simulink model "dsPIC33CK256MP508_MCLV2_SMO"  (R2021b)
settings: Solver=FixedStepDiscrete  StartTime=0.0  StopTime=10  FixedStep=.00005  RelTol=1e-3  EnableMultiTasking=on
PreLoadFcn:
  | dsPIC33CK256MP508_MCLV2_SMO_data;
InitFcn:
  | dsPIC33CK256MP508_MCLV2_SMO_data;
undefined symbols (not defined in the file): AN1, B0, B2, C9, D6, DiscIntNeverNeededParam, inverter, MaxPer, mcb_isCodeGenVar, mcb_isSimVar, P32, P57, P70, PI_params, Pin, pmsm, PU_System, PWM1max, PWM_frequency, Resol, s, Speed_openLoop, Ts, Ts_speed, us
libraries: mcbcontrolslib x13, MCHP_Blockset x13, simulink x10, mcbplantlib x1, autolibpmsmexterior x1
(part 2 of 3)

== system dsPIC33CK256MP508_MCLV2_SMO/Current Control/MOTOR Cmd ==
  PWM (abc) : Inport
  Dead time Compensation : Bias  Bias=round( (2e-6/5e-5) *PWM1max )
  Demux : Demux  Outputs=3
  PWM_HS_FEP : MCHP_Blockset/PWM IO/PWM_HS_FEP  Priority=-2000  PWMx_MODSEL=Center Aligned  PWMx_CLKSEL=no scaling  PWM_ClockResolution_DIVSEL=Dynamic Options  PWM_ClockResolution_DIVSEL_TXT=auto  PWM_ClockResolution_FSCL=Dynamic Options  PWM_ClockResolution_FSCL_TXT=auto - no jitter  PWM_ClockResolution_NoScaling=Dynamic Options  PWM_ClockResolution_NoScaling_TXT="Resol: 0.005(us)  -  MaxPer: 0.000328(s)"  MaxPeriod_s=50e-6  InitPeriode_s=50e-6  InitDutyCycleP_s=2e-6  InitDutyCycleS_s=10e-6  InitPhase_s=-1  evalin_ws=PWM1max=MCHP_Fun.Hex2num('40B3880000000000');PWM2max=MCHP_Fun.Hex2num('40B3880000000000');PWM3max=MCHP_Fun.Hex2num('40B3880000000000');  SampleTime=-1  S_INPUT=[-1]  S_INPUT_Size=[3]  S_OUTPUT=[]  S_OUTPUT_Size=[]  S_ListCustomDatatype=S.S_ListCustomDatatype={};  MCHP_USER_INTERRUPTS=0  MCHP_PORT={PWMH1 }{PWMH1}32:4:B14;{PWMH2 }{PWMH2}32:4:B12;{PWMH3 }{PWMH3}32:4:B10;{PWML1}{PWML1}32:4:B15;{PWML2}{PWML2}32:4:B13;{PWML3}{PWML3}32:4:B11;  MCHP_MASTERLINK=dsPIC33CK256MP508_MCLV2_SMO1/Hardware Init/Microchip Master  MCHP_CRC=4827838  PWMx_PMOD=Complementary  PWM1_HL=PWMxH & PWMxL output enabled  PWM1_swap=off  PWM1H_pol=off  PWM1L_pol=off  PWM2_HL=PWMxH & PWMxL output enabled  PWM2_swap=off  PWM2H_pol=off  PWM2L_pol=off  PWM3_HL=PWMxH & PWMxL output enabled  PWM3_swap=off  PWM3H_pol=off  PWM3L_pol=off  PWM4_HL=not used  PWM4_swap=off  PWM4H_pol=off  PWM4L_pol=off  PWM5_HL=not used  PWM5_swap=off  PWM5H_pol=off  PWM5L_pol=off  PWM6_HL=not used  PWM6_swap=off  PWM6H_pol=off  PWM6L_pol=off  PWM7_HL=not used  PWM7_swap=off  PWM7H_pol=off  PWM7L_pol=off  PWM8_HL=not used  PWM8_swap=off  PWM8H_pol=off  PWM8L_pol=off  PWM9_HL=not used  PWM9_swap=off  PWM9H_pol=off  PWM9L_pol=off  PWM10_HL=not used  PWM10_swap=off  PWM10H_pol=off  PWM10L_pol=off  PWM11_HL=not used  PWM11_swap=off  PWM11H_pol=off  PWM11L_pol=off  PWM12_HL=not used  PWM12_swap=off  PWM12H_pol=off  PWM12L_pol=off  PWM1_ShowTrig=on  PWM1_Init_PGxTRIGABC_s=[0 -1 -1 ]  PWM1_ADTRxEN1=ADC Trigger 1  PWM1_ADTRxEN2=none  PWM1_ADTRxEN3=none  PWM2_ShowTrig=off  PWM2_Init_PGxTRIGABC_s=[-1 -1 -1]  PWM2_ADTRxEN1=none  PWM2_ADTRxEN2=none  PWM2_ADTRxEN3=none  PWM3_ShowTrig=off  PWM3_Init_PGxTRIGABC_s=[-1 -1 -1]  PWM3_ADTRxEN1=none  PWM3_ADTRxEN2=none  PWM3_ADTRxEN3=none  PWM4_ShowTrig=off  PWM4_Init_PGxTRIGABC_s=[-1 -1 -1]  PWM4_ADTRxEN1=none  PWM4_ADTRxEN2=none  PWM4_ADTRxEN3=none  PWM5_ShowTrig=off  PWM5_Init_PGxTRIGABC_s=[-1 -1 -1]  PWM5_ADTRxEN1=none  PWM5_ADTRxEN2=none  PWM5_ADTRxEN3=none  PWM6_ShowTrig=off  PWM6_Init_PGxTRIGABC_s=[-1 -1 -1]  PWM6_ADTRxEN1=none  PWM6_ADTRxEN2=none  PWM6_ADTRxEN3=none  PWM7_ShowTrig=off  PWM7_Init_PGxTRIGABC_s=[-1 -1 -1]  PWM7_ADTRxEN1=none  PWM7_ADTRxEN2=none  PWM7_ADTRxEN3=none  PWM8_ShowTrig=off  PWM8_Init_PGxTRIGABC_s=[-1 -1 -1]  PWM8_ADTRxEN1=none  PWM8_ADTRxEN2=none  PWM8_ADTRxEN3=none  BlockInput_VectorScalar=Independant Scalar  BlockInput_Period=Not a block input  BlockInput_DutyCycle=a Uint raw input (PWMxmax variable represent max period)  BlockInput_PhaseShift=Not a block input  BlockInput_SEVTCMP=Not a block input  BlockInput_TRIGx=Not a block input  BlockInput_DeadTime=Not a block input  BlockOutput_FaultDisabled=off  BlockOutput_Fault=on  DTC=Positive dead time (ensure period of time with PWM_H and PWM_L disasserted)  FLTSRC1_DTCMP=Dynamic Options  FLTSRC1_DTCMP_TXT=<empty>  FLTSRC2_DTCMP=Dynamic Options  FLTSRC2_DTCMP_TXT=<empty>  FLTSRC3_DTCMP=Dynamic Options  FLTSRC3_DTCMP_TXT=<empty>  FLTSRC4_DTCMP=Dynamic Options  FLTSRC4_DTCMP_TXT=<empty>  FLTSRC5_DTCMP=Dynamic Options  FLTSRC5_DTCMP_TXT=<empty>  FLTSRC6_DTCMP=Dynamic Options  FLTSRC6_DTCMP_TXT=<empty>  FLTSRC7_DTCMP=Dynamic Options  FLTSRC7_DTCMP_TXT=<empty>  FLTSRC8_DTCMP=Dynamic Options  FLTSRC8_DTCMP_TXT=<empty>  FLTSRC9_DTCMP=Dynamic Options  FLTSRC9_DTCMP_TXT=<empty>  FLTSRC10_DTCMP=Dynamic Options  FLTSRC10_DTCMP_TXT=<empty>  FLTSRC11_DTCMP=Dynamic Options  FLTSRC11_DTCMP_TXT=<empty>  FLTSRC12_DTCMP=Dynamic Options  FLTSRC12_DTCMP_TXT=<empty>  DeadTime_s=1e-6  DeadTimeAlt_s=1e-6  DeadTimeComp_s=0  FLTMODx=Disabled  FLTSRCx=Dynamic Options  FLTSRCx_TXT=<empty>  FLTDATx=PWM H/L -> 11  CLMODx=Disabled  CLSRCx=Dynamic Options  CLSRCx_TXT=<empty>  CLDATx=PWM H/L -> 00  FLTLEBENx=off  CLLEBENx=off  LeadEdgeBlkPer_s=5e-7  PHRx=off  PHFx=off  PLRx=off  PLFx=off
      settings: SourceProductName=MPLAB Device Blocks for Simulink
  "Saturation " : Saturate  UpperLimit=PWM1max  LowerLimit=round( (2e-6/5e-5) *PWM1max )* 2
  int to uint : DataTypeConversion  OutDataTypeStr=uint16  ConvertRealWorld=Stored Integer (SI)
  tag scope: Duty1=global
  wires:
  int to uint/1 -> "Saturation "/1
  Dead time Compensation/1 -> [Duty1], int to uint/1
  PWM (abc)/1 -> Dead time Compensation/1
  "Saturation "/1 -> Demux/1
  Demux/2 -> PWM_HS_FEP/2
  Demux/3 -> PWM_HS_FEP/3
  Demux/1 -> PWM_HS_FEP/1

== system dsPIC33CK256MP508_MCLV2_SMO/Current Control/MOTOR - Board Sensor ==
  ADC dsPIC High Speed SAR : MCHP_Blockset/Analog IO/ADC dsPIC High Speed SAR  ACLKCON=Not used  ADC_FRACT=Fractional (left aligned)  ADC_NRE=off  DMA_Size=Single trigger - (default)  ADC_Synchronisation=Triggered by custom source  ADC_Trig=Dynamic Options  ADC_Trig_TXT=PWM1 Trigger 1  ADC_TrigTimeStep=Trig model step after all sample from this block are converted  ADC_TrigInfo=0  SampleTime=Ts  S_INPUT=[]  S_INPUT_Size=[]  S_OUTPUT="[5  5]"  S_OUTPUT_Size="[1  1]"  S_ListCustomDatatype=S.S_ListCustomDatatype={};  MCHP_USER_INTERRUPTS={ADCAN1}{ADCBUF1}{ADC Data 1 Ready}{VectorName(ADCAN1Interrupt) Priority(-1) RegisterReadClear(ADCBUF1)Config_BitSet(ADIELbits.IE1) };{ADCAN3}{ADCBUF3}{ADC Data 3 Ready}{VectorName(ADCAN3Interrupt) Priority(-1) RegisterReadClear(ADCBUF3)Config_BitSet(ADIELbits.IE3) };{ADCAN18}{ADCBUF18}{ADC Data 18 Ready}{VectorName(ADCAN18Interrupt) Priority(-1) RegisterReadClear(ADCBUF18)Config_BitSet(ADIEHbits.IE18) };  MCHP_PORT={Analog Input 1}{AN1}15:2:B2;{Analog Input 4}{AN4}15:2:A4;{Analog Input 19}{AN19}15:2:D11;  MCHP_MASTERLINK=dsPIC33CK256MP508_MCLV2_SMO1/Hardware Init/Microchip Master  MCHP_CRC=4003151  ADC_Info=Total Time = 4.92(us)  ADC0_pin=Dynamic Options  ADC0_pin_TXT=Not used  ADC0_R="< 50   kOhm"  ADC0_res=12 bits  ADC0_signed=signed 16 bits  ADC0_FILTER=No Oversampling  ADC0_FILTER_nSamples=256 samples  ADC0_STRGEN=Start sampling followed by conversion  ADC0_STRGEN_on=Start sampling followed by conversion  ADC0_SSAMPEN=off  ADC0_Info=tSmp_min=20(ns) x 0 = 0(s) ; tConv=210(ns) x 0 = 0(s) ; TOTAL=0(s)  ADC1_pin=Dynamic Options  ADC1_pin_TXT=AN1 / B2 / Pin[41]  ADC1_R="< 50   kOhm"  ADC1_res=12 bits  ADC1_signed=signed 16 bits  ADC1_FILTER=No Oversampling  ADC1_FILTER_nSamples=128 samples  ADC1_STRGEN=Start sampling followed by conversion  ADC1_STRGEN_on=Start sampling followed by conversion  ADC1_SSAMPEN=off  ADC1_Info=tSmp_min=2.06(us) x 1 = 2.06(us) ; tConv=370(ns) x 1 = 370(ns) ; TOTAL=2.44(us)  ADC2_pin=Dynamic Options  ADC2_pin_TXT=Not used  ADC2_R="< 5    kOhm"  ADC2_res=12 bits  ADC2_signed=signed 16 bits  ADC2_FILTER=No Oversampling  ADC2_FILTER_nSamples=256 samples  ADC2_STRGEN=End sampling and start conversion  ADC2_STRGEN_on=Start sampling followed by conversion  ADC2_SSAMPEN=on  ADC2_Info=tSmp_min=14.706(ns) x 0 = 0(s) ; tConv=154.41(ns) x 0 = 0(s) ; TOTAL=0(s)  ADC3_pin=Dynamic Options  ADC3_pin_TXT=Not used  ADC3_R="< 10   kOhm"  ADC3_res=12 bits  ADC3_signed=signed 16 bits  ADC3_FILTER=Burst convert of n samples are Summed  ADC3_FILTER_nSamples=64 samples  ADC3_STRGEN=End sampling and start conversion  ADC3_STRGEN_on=Start sampling followed by conversion  ADC3_SSAMPEN=on  ADC3_Info=tSmp_min=14.706(ns) x 0 = 0(s) ; tConv=154.41(ns) x 0 = 0(s) ; TOTAL=0(s)  ADC4_pin=Dynamic Options  ADC4_pin_TXT=Not used  ADC4_R=< 200 Ohm  ADC4_res=12 bits  ADC4_signed=unsigned 16 bits  ADC4_FILTER=No Oversampling  ADC4_FILTER_nSamples=256 samples  ADC4_STRGEN=End sampling and start conversion  ADC4_STRGEN_on=Start sampling followed by conversion  ADC4_SSAMPEN=off  ADC4_Info=tSmp_min=14.706(ns) x 0 = 0(s) ; tConv=154.41(ns) x 0 = 0(s) ; TOTAL=0(s)  ADC5_pin=Dynamic Options  ADC5_pin_TXT=Not used  ADC5_R=< 200 Ohm  ADC5_res=12 bits  ADC5_signed=unsigned 16 bits  ADC5_FILTER=Burst convert of n samples are Summed  ADC5_FILTER_nSamples=256 samples  ADC5_STRGEN=End sampling and start conversion  ADC5_STRGEN_on=Start sampling followed by conversion  ADC5_SSAMPEN=on  ADC5_Info=tSmp_min=14.706(ns) x 0 = 0(s) ; tConv=154.41(ns) x 0 = 0(s) ; TOTAL=0(s)  ADC6_pin=Dynamic Options  ADC6_pin_TXT=Not used  ADC6_R=< 200 Ohm  ADC6_res=12 bits  ADC6_signed=unsigned 16 bits  ADC6_FILTER=Burst convert of n samples are Summed  ADC6_FILTER_nSamples=256 samples  ADC6_STRGEN=End sampling and start conversion  ADC6_STRGEN_on=Start sampling followed by conversion  ADC6_SSAMPEN=on  ADC6_Info=tSmp_min=14.706(ns) x 0 = 0(s) ; tConv=154.41(ns) x 0 = 0(s) ; TOTAL=0(s)  ADC7_R="< 50   kOhm"  ADC7_res=12 bits  ADC7_AN0=Not used  ADC7_AN1=Not used  ADC7_AN2=Not used  ADC7_AN3=Not used  ADC7_AN4=signed int16  ADC7_AN5=Not used  ADC7_AN6=Not used  ADC7_AN7=Not used  ADC7_AN8=Not used  ADC7_AN9=Not used  ADC7_AN10=Not used  ADC7_AN11=Not used  ADC7_AN12=Not used  ADC7_AN13=Not used  ADC7_AN14=Not used  ADC7_AN15=Not used  ADC7_AN16=Not used  ADC7_AN17=Not used  ADC7_AN18=Not used  ADC7_AN19=unsigned int16  ADC7_AN20=Not used  ADC7_AN21=Not used  ADC7_AN22=Not used  ADC7_AN23=Not used  ADC7_AN24=Not used  ADC7_AN25=Not used  ADC7_AN26=Not used  ADC7_AN27=Not used  ADC7_AN28=Not used  ADC7_AN29=Not used  ADC7_AN30=Not used  ADC7_AN31=Not used  IVref=Not used  IVTemp=Not used  ADC7_Info=tSmp_min=2.08(us) x 2 = 4.16(us) ; tConv=370(ns) x 2 = 740(ns) ; TOTAL=4.92(us)
      settings: SourceProductName=MPLAB Device Blocks for Simulink
  Add2 : Sum  Inputs=+-  OutDataTypeStr=int16  RndMeth=Simplest
  Data Store Read : DataStoreRead  DataStoreName=EnCurOffset  IndexOptions=Index vector (dialog)  Indices=1  OutputSizes=1
  Data Type Conversion : DataTypeConversion  OutDataTypeStr=dataType  RndMeth=Simplest
  Gain Correction : Subsystem
  Mux2 : Mux  Inputs=2
  Offset1 : Subsystem
  Q1.15 : DataTypeConversion  OutDataTypeStr=fixdt(0,16,16)  ConvertRealWorld=Stored Integer (SI)
  Scale Ia Ib to (A) : DataTypeConversion  OutDataTypeStr=fixdt(1,16, 1.65/32768 / (.005 * 75),0)  ConvertRealWorld=Stored Integer (SI)
  Pot : Outport  VectorParamsAs1DForOutWhenUnconnected=off
  Iab (A) : Outport  Port=2  VectorParamsAs1DForOutWhenUnconnected=off
  tag scope: Iab=global, Pot=global
  wires:
  Mux2/1 -> Add2/1, Offset1/1(Iab)
  ADC dsPIC High Speed SAR/3 -> Q1.15/1  "U2 CH2"
  Q1.15/1 -> Data Type Conversion/1
  Scale Ia Ib to (A)/1 -> Gain Correction/1(In1)  "Ia Ib"
  Offset1/1(Offset) -> Add2/2
  Add2/1 -> Scale Ia Ib to (A)/1
  Data Store Read/1 -> Offset1/Enable
  Data Type Conversion/1 -> Pot/1, [Pot]
  Gain Correction/1(Out1) -> Iab (A)/1, [Iab]
  ADC dsPIC High Speed SAR/1 -> Mux2/1
  ADC dsPIC High Speed SAR/2 -> Mux2/2

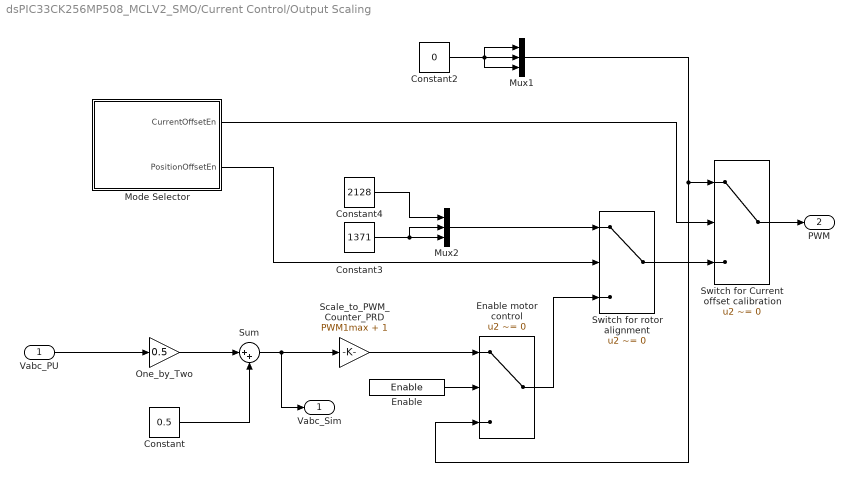
== system dsPIC33CK256MP508_MCLV2_SMO/Current Control/Output Scaling ==
  Vabc_PU : Inport
  Constant : Constant  Value=0.5  OutDataTypeStr=dataType  SampleTime=-1
  Constant2 : Constant  Value=0  OutDataTypeStr=Inherit: Inherit via back propagation
  Constant3 : Constant  Value=1371  OutDataTypeStr=Inherit: Inherit via back propagation
  Constant4 : Constant  Value=2128  OutDataTypeStr=Inherit: Inherit via back propagation
  Enable : DataStoreRead  DataStoreName=Enable  IndexOptions=Index vector (dialog)  Indices=1  OutputSizes=1
  Enable motor control : Switch  Criteria=u2 ~= 0  Threshold=250
  Mode Selector : Subsystem
  Mux1 : Mux  Inputs=3
  Mux2 : Mux  Inputs=3
  One_by_Two : Gain  Gain=0.5  RndMeth=Simplest  OutDataTypeStr=Inherit: Same as input
  Scale_to_PWM_Counter_PRD : Gain  Gain=PWM1max + 1  OutDataTypeStr=uint16  RndMeth=Simplest
  Sum : Sum  Inputs=|++
  Switch for Current offset calibration : Switch  Criteria=u2 ~= 0  Threshold=250
  Switch for rotor alignment : Switch  Criteria=u2 ~= 0  Threshold=250
  Vabc_Sim : Outport
  PWM : Outport  Port=2
  wires:
  Sum/1 -> Scale_to_PWM_Counter_PRD/1, Vabc_Sim/1
  Constant/1 -> Sum/2
  Switch for Current offset calibration/1 -> PWM/1
  One_by_Two/1 -> Sum/1
  Switch for rotor alignment/1 -> Switch for Current offset calibration/3
  Scale_to_PWM_Counter_PRD/1 -> Enable motor control/1
  Vabc_PU/1 -> One_by_Two/1
  Mode Selector/2(PositionOffsetEn) -> Switch for rotor alignment/2
  Mux2/1 -> Switch for rotor alignment/1
  Mux1/1 -> Enable motor control/3, Switch for Current offset calibration/1
  Constant2/1 -> Mux1/1, Mux1/3, Mux1/2
  Constant3/1 -> Mux2/3, Mux2/2
  Constant4/1 -> Mux2/1
  Mode Selector/1(CurrentOffsetEn) -> Switch for Current offset calibration/2
  Enable/1 -> Enable motor control/2
  Enable motor control/1 -> Switch for rotor alignment/3

== system dsPIC33CK256MP508_MCLV2_SMO/Current Control/Serial Tx ==
  Data : Inport
  Counter Limited : simulink/Sources/Counter Limited  uplimit=3  tsamp=-1
  Data Type Conversion : DataTypeConversion  OutDataTypeStr=uint8  RndMeth=Simplest
  Demux : Demux
  Index Vector : MultiPortSwitch  DataPortOrder=Zero-based contiguous  Inputs=4  zeroidx=on  OutDataTypeStr=Inherit: Same as first data input  RndMeth=Simplest
  UART_TX : Subsystem
  wires:
  Data Type Conversion/1 -> UART_TX/1(Count), Index Vector/1
  Index Vector/1 -> UART_TX/2(Data)
  Demux/4 -> Index Vector/5
  Demux/3 -> Index Vector/4
  Demux/1 -> Index Vector/2
  Demux/2 -> Index Vector/3
  Data/1 -> Demux/1
  Counter Limited/1 -> Data Type Conversion/1

== system dsPIC33CK256MP508_MCLV2_SMO/Hardware Init/Open Board and Motor pages ==

== system dsPIC33CK256MP508_MCLV2_SMO/Inverter and Motor/Codegeneration ==
  Duty_Cycles : Inport
  Ground : Ground
  Terminator : Terminator
  Feedbacks_Iab : Outport  VectorParamsAs1DForOutWhenUnconnected=off
  wires:
  Ground/1 -> Feedbacks_Iab/1
  Duty_Cycles/1 -> Terminator/1

== system dsPIC33CK256MP508_MCLV2_SMO/Inverter and Motor/Simulation ==
  Duty_Cycles : Inport
  Gain9 : Gain  Gain=(60/(2*pi))/PU_System.N_base
  Inverter : Subsystem
  Load_Profile (Torque) : Subsystem
  Scope : Scope
  Scope1 : Scope
  Scope2 : Scope
  Sensor_Measurements : Subsystem
  Surface Mount PMSM : autolibpmsmexterior/Surface Mount PMSM  port_config=Torque  sim_type=Discrete  Ts=Ts  P=pmsm.p  Rs=pmsm.Rs + inverter.R_board  Ldq_=pmsm.Ld  KConstText=Permanent flux linkage constant (lambda_pm):  lambda_pm=pmsm.FluxPM  Ke=159.9771  Kt=1.323  mechanical=[pmsm.J, pmsm.B, 0]  idq0=[0 0]  theta_init=0  omega_init=0  KConst=pmsm.FluxPM  lambda_pm_calc=pmsm.FluxPM  RefBlkName='autolibpmsmexterior/Surface Mount PMSM'  aMode=5  Ldq="[0.0002      0.0002]"
      settings: SourceProductBaseCode=PW,DR,MT,UV,VE
  Terminator : Terminator
  Terminator1 : Terminator
  Feedbacs_Iab : Outport  VectorParamsAs1DForOutWhenUnconnected=off
  wires:
  Surface Mount PMSM/1 -> Sensor_Measurements/1(Info)
  Duty_Cycles/1 -> Scope2/1, Inverter/1(Duty_abc)
  Surface Mount PMSM/2 -> Sensor_Measurements/2(PhaseCurr)  "Iabc"
  Sensor_Measurements/1(Iab_fb) -> Scope/1, Feedbacs_Iab/1
  Load_Profile (Torque)/1(Load_Trq) -> Surface Mount PMSM/1
  Inverter/1(Vabc) -> Scope1/1, Surface Mount PMSM/2
  Sensor_Measurements/2(Pos_fb) -> Terminator1/1
  Gain9/1 -> Terminator/1
  Surface Mount PMSM/3 -> Gain9/1

== system dsPIC33CK256MP508_MCLV2_SMO/Speed Control/Enable Switch ==
  Codegen : Subsystem  VariantControl=mcb_isCodeGenVar()
  Sim : Subsystem  VariantControl=mcb_isSimVar()

== system dsPIC33CK256MP508_MCLV2_SMO/Speed Control/PI_Controller_Speed ==
  N_ref : Inport
  N_fb : Inport  Port=2
  Data Store Read1 : DataStoreRead  DataStoreName=EnSpeedCtrl  IndexOptions=Index vector (dialog)  Indices=1  OutputSizes=1
  Discrete PI Controller with anti-windup & reset : mcbcontrolslib/Discrete PI Controller  with anti-windup & reset  UpperSaturationLimit=1  LowerSaturationLimit=-1
      settings: SourceProductBaseCode=MT
  Ki1 : Constant  Value=PI_params.Ki_speed*Ts_speed  OutDataTypeStr=dataType  SampleTime=-1
  Ki2 : Constant  Value=0  OutDataTypeStr=dataType  SampleTime=-1
  Kp1 : Constant  Value=PI_params.Kp_speed  OutDataTypeStr=dataType  SampleTime=-1
  Logical Operator : Logic  Operator=NOT  IconShape=distinctive  AllPortsSameDT=off  OutDataTypeStr=boolean
  Scope : Scope
  Sum : Sum  Inputs=|+-  OutDataTypeStr=Inherit: Same as first input
  Zero_Cancellation : mcbcontrolslib/IIR Filter  VariantControl=Low Pass Filter  VariantSelect=Low-pass  Filter_constant=0.001*(Ts_speed/Ts)  advancedSettings=off  Ts=50e-6  cutOff_freq=98.4464
      settings: SourceProductBaseCode=MT
  Iq_ref : Outport  VectorParamsAs1DForOutWhenUnconnected=off
  wires:
  Discrete PI Controller with anti-windup & reset/1 -> Iq_ref/1
  Ki1/1 -> Discrete PI Controller with anti-windup & reset/3
  Kp1/1 -> Discrete PI Controller with anti-windup & reset/2
  N_fb/1 -> Sum/2
  N_ref/1 -> Zero_Cancellation/1
  Sum/1 -> Discrete PI Controller with anti-windup & reset/1
  Logical Operator/1 -> Scope/1, Discrete PI Controller with anti-windup & reset/4
  Ki2/1 -> Discrete PI Controller with anti-windup & reset/5
  Data Store Read1/1 -> Logical Operator/1
  Zero_Cancellation/1 -> Sum/1

== system dsPIC33CK256MP508_MCLV2_SMO/Speed Control/Speed_Ref_Selector ==
  Speed_Ref_In : Inport
  Constant : Constant  Value=0  OutDataTypeStr=dataType
  Data Store Read1 : DataStoreRead  DataStoreName=EnableFOC  IndexOptions=Index vector (dialog)  Indices=1  OutputSizes=1
  Switch : Switch  Criteria=u2 > Threshold  Threshold=0.5
  Speed_Ref_PU : Outport
  wires:
  Switch/1 -> Speed_Ref_PU/1
  Constant/1 -> Switch/3
  Speed_Ref_In/1 -> Switch/1
  Data Store Read1/1 -> Switch/2

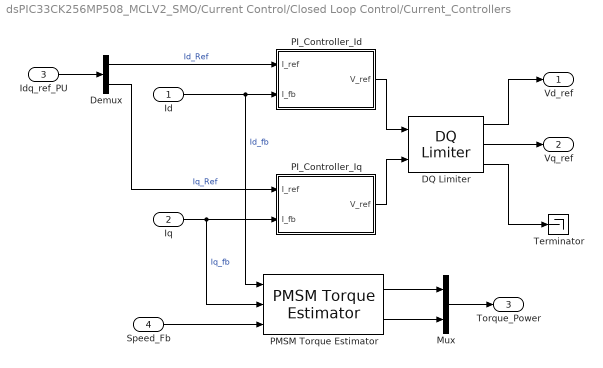
== system dsPIC33CK256MP508_MCLV2_SMO/Current Control/Closed Loop Control/Current_Controllers ==
  Id : Inport
  Iq : Inport  Port=2
  Idq_ref_PU : Inport  Port=3
  Speed_Fb : Inport  Port=4
  DQ Limiter : mcbcontrolslib/DQ Limiter  Vmax=0.95
      settings: SourceProductBaseCode=MT
  Demux : Demux  Outputs=2
  Mux : Mux  Inputs=2
  PI_Controller_Id : Subsystem
  PI_Controller_Iq : Subsystem
  PMSM Torque Estimator : mcbcontrolslib/PMSM Torque Estimator  polePairs=pmsm.p  Ld=pmsm.Ld  Lq=pmsm.Lq  FluxPM=pmsm.FluxPM  Units=Per-Unit (PU)  V_base=PU_System.V_base  I_base=PU_System.I_base  N_base=PU_System.N_base  T_base=0.26718  P_base=91.4523
      settings: SourceProductBaseCode=MT
  Terminator : Terminator
  Vd_ref : Outport  VectorParamsAs1DForOutWhenUnconnected=off
  Vq_ref : Outport  Port=2  VectorParamsAs1DForOutWhenUnconnected=off
  Torque_Power : Outport  Port=3
  wires:
  Iq/1 -> PMSM Torque Estimator/2, PI_Controller_Iq/2(I_fb)  "Iq_fb"
  Id/1 -> PMSM Torque Estimator/1, PI_Controller_Id/2(I_fb)  "Id_fb"
  Demux/1 -> PI_Controller_Id/1(I_ref)  "Id_Ref"
  Demux/2 -> PI_Controller_Iq/1(I_ref)  "Iq_Ref"
  Idq_ref_PU/1 -> Demux/1
  PI_Controller_Id/1(V_ref) -> DQ Limiter/1
  PI_Controller_Iq/1(V_ref) -> DQ Limiter/2
  DQ Limiter/1 -> Vd_ref/1
  DQ Limiter/2 -> Vq_ref/1
  DQ Limiter/3 -> Terminator/1
  PMSM Torque Estimator/1 -> Mux/1
  PMSM Torque Estimator/2 -> Mux/2
  Mux/1 -> Torque_Power/1
  Speed_Fb/1 -> PMSM Torque Estimator/3

== system dsPIC33CK256MP508_MCLV2_SMO/Current Control/Input Scaling/OpenLoopTheta ==
  Enable : EnablePort
  Constant : Constant  Value=500/PU_System.N_base  OutDataTypeStr=dataType
  Data Type Conversion : DataTypeConversion  OutDataTypeStr=fixdt(1,32,20)  ConvertRealWorld=Stored Integer (SI)
  Discrete-Time Integrator : DiscreteIntegrator  IntegratorMethod=Accumulation: Forward Euler  gainval=0.002  SampleTime=Ts  OutDataTypeStr=fixdt(1,32,20)  LimitOutput=on  UpperSaturationLimit=500/PU_System.N_base  LowerSaturationLimit=0  ICPrevOutput=DiscIntNeverNeededParam  ICPrevScaledInput=DiscIntNeverNeededParam
  Gain : Gain  Gain=Ts*PU_System.N_base*pmsm.p/60  OutDataTypeStr=dataType  ParamDataTypeStr=Inherit: Same as input
  Position Generator : mcbcontrolslib/Position Generator  AngleOutput=Per-unit  ThetaSource=External  ThetaInput=5e-4  DataType=double  ExternalReset=none  Offset=0
      settings: SourceProductBaseCode=MT
  Scope : Scope
  eps : Outport
  wires:
  Gain/1 -> Position Generator/1
  Constant/1 -> Data Type Conversion/1
  Data Type Conversion/1 -> Discrete-Time Integrator/1
  Position Generator/1 -> Scope/1, eps/1
  Discrete-Time Integrator/1 -> Gain/1

== system dsPIC33CK256MP508_MCLV2_SMO/Current Control/Input Scaling/OpentoClosed ==
  Speed_fb : Inport
  Chart : Stateflow chart  TreatAsAtomicUnit=on
  Data Store Read5 : DataStoreRead  DataStoreName=Enable  IndexOptions=Index vector (dialog)  Indices=1  OutputSizes=1
  Data Store Write1 : DataStoreWrite  DataStoreName=EnSpeedCtrl  IndexOptions=Index vector (dialog)  Indices=1  OutputSizes=1
  Data Store Write2 : DataStoreWrite  DataStoreName=EnableClosedLoop  IndexOptions=Index vector (dialog)  Indices=1  OutputSizes=1
  Data Type Conversion : DataTypeConversion  OutDataTypeStr=boolean  RndMeth=Simplest
  Data Type Conversion1 : DataTypeConversion  OutDataTypeStr=boolean
  Enable Closed Loop : Constant  OutDataTypeStr=uint16
  Enable Closed Loop1 : Constant  Value=Speed_openLoop/PU_System.N_base  OutDataTypeStr=dataType
  Open Loop Start-up : Constant  Value=0  OutDataTypeStr=uint16
  Switch2 : Switch  Criteria=u2 > Threshold  Threshold=1
  EnClosedLoop : Outport
  wires:
  Open Loop Start-up/1 -> Switch2/3
  Data Store Read5/1 -> Chart/3(En)
  Chart/1(Mode) -> Switch2/2
  Switch2/1 -> Data Type Conversion/1
  Speed_fb/1 -> Chart/2(SpeedFb)
  Enable Closed Loop/1 -> Switch2/1
  Enable Closed Loop1/1 -> Chart/1(Limit)
  Data Type Conversion/1 -> EnClosedLoop/1, Data Store Write2/1
  Chart/2(SpeedCtrl) -> Data Type Conversion1/1
  Data Type Conversion1/1 -> Data Store Write1/1

== system dsPIC33CK256MP508_MCLV2_SMO/Current Control/Input Scaling/Sliding Mode Observer ==
  Ialpha_PU : Inport
  Ibeta_PU : Inport  Port=2
  Valpha_PU : Inport  Port=3
  Vbeta_PU : Inport  Port=4
  SpeedRef_PU : Inport  Port=5
  Scaling : Subsystem
  smo : Subsystem
  theta : Outport
  west : Outport  Port=2
  wires:
  Scaling/1(Ialpha) -> smo/1(ialfa)
  Scaling/5(SpeedRef) -> smo/5(wref)
  Valpha_PU/1 -> Scaling/3(Valpha_PU)
  Scaling/4(Vbeta) -> smo/4(vbeta)
  Scaling/2(Ibeta) -> smo/2(ibeta)
  Scaling/3(Valpha) -> smo/3(valfa)
  smo/2(west) -> west/1
  SpeedRef_PU/1 -> Scaling/5(SpeedRef_PU)
  smo/1(theta) -> theta/1
  Vbeta_PU/1 -> Scaling/4(Vbeta_PU)
  Ibeta_PU/1 -> Scaling/2(Ibeta_PU)
  Ialpha_PU/1 -> Scaling/1(Ialpha_PU)

== system dsPIC33CK256MP508_MCLV2_SMO/Current Control/MOTOR - Board Sensor/Gain Correction ==
  In1 : Inport
  Demux : Demux  Outputs=2
  Gain : Gain  Gain=0.865  RndMeth=Zero  OutDataTypeStr=Inherit: Same as input
  Gain1 : Gain  Gain=0.961  RndMeth=Zero  OutDataTypeStr=Inherit: Same as input
  Mux : Mux  Inputs=2
  To Per-Unit : Gain  Gain=inverter.invertingAmp/PU_System.I_base  OutMin=-1  OutMax=1  OutDataTypeStr=fixdt(1,16)  RndMeth=Zero
  Out1 : Outport
  wires:
  Demux/1 -> Gain/1
  To Per-Unit/1 -> Demux/1
  Gain/1 -> Mux/1
  Mux/1 -> Out1/1
  In1/1 -> To Per-Unit/1
  Demux/2 -> Gain1/1
  Gain1/1 -> Mux/2

== system dsPIC33CK256MP508_MCLV2_SMO/Current Control/MOTOR - Board Sensor/Offset1 ==
  Iab : Inport
  Enable : EnablePort
  Offset : Outport
  wires:
  Iab/1 -> Offset/1

== system dsPIC33CK256MP508_MCLV2_SMO/Current Control/Output Scaling/Mode Selector ==
  Delay : Delay  DelayLength=1
  NOT : Logic  Operator=NOT  IconShape=distinctive  AllPortsSameDT=off  OutDataTypeStr=boolean
  Subsystem1 : Subsystem
  Up Counter : Subsystem
  CurrentOffsetEn : Outport
  PositionOffsetEn : Outport  Port=2
  wires:
  Up Counter/1(Count) -> Subsystem1/1(Count)
  Delay/1 -> NOT/1
  NOT/1 -> Up Counter/Enable
  Subsystem1/1(Current Offset) -> CurrentOffsetEn/1
  Subsystem1/2(PositionOffset) -> PositionOffsetEn/1
  Subsystem1/3(EnableFOC) -> Delay/1

== system dsPIC33CK256MP508_MCLV2_SMO/Current Control/Serial Tx/UART_TX ==
  Count : Inport
  Data : Inport  Port=2
  Debug_Data : Subsystem
  SCI_Tx : Subsystem
  wires:
  Count/1 -> Debug_Data/1(Count)
  Debug_Data/1(Data_log) -> SCI_Tx/1(Data_Log)
  Data/1 -> Debug_Data/2(Data)

== system dsPIC33CK256MP508_MCLV2_SMO/Inverter and Motor/Simulation/Inverter ==
  Duty_abc : Inport
  Average-Value Inverter : mcbplantlib/Average-Value Inverter
  Constant2 : Constant  Value=inverter.V_dc  OutDataTypeStr=single  SampleTime=-1
  Data Type Conversion1 : DataTypeConversion  OutDataTypeStr=single  RndMeth=Simplest
  Vabc : Outport  VectorParamsAs1DForOutWhenUnconnected=off
  wires:
  Average-Value Inverter/1 -> Vabc/1
  Data Type Conversion1/1 -> Average-Value Inverter/1
  Duty_abc/1 -> Data Type Conversion1/1
  Constant2/1 -> Average-Value Inverter/2

== system dsPIC33CK256MP508_MCLV2_SMO/Inverter and Motor/Simulation/Load_Profile (Torque) ==
  Data Type Conversion : DataTypeConversion  OutDataTypeStr=single
  IIR Filter : mcbcontrolslib/IIR Filter  VariantControl=Low Pass Filter  VariantSelect=Low-pass  Filter_constant=0.01  advancedSettings=off  Ts=50e-6  cutOff_freq=32.1525
      settings: SourceProductBaseCode=MT
  Step : Step  Time=8  Before=0.0* pmsm.T_rated  After=0.1* pmsm.T_rated
  Load_Trq : Outport  VectorParamsAs1DForOutWhenUnconnected=off
  wires:
  IIR Filter/1 -> Load_Trq/1
  Data Type Conversion/1 -> IIR Filter/1
  Step/1 -> Data Type Conversion/1

== system dsPIC33CK256MP508_MCLV2_SMO/Inverter and Motor/Simulation/Sensor_Measurements ==
  note: Delays
  note: Scaling
  Info : Inport
  PhaseCurr : Inport  Port=2
  Bus Selector : BusSelector  OutputSignals=MtrPos
  Data Type Conversion2 : DataTypeConversion  OutDataTypeStr=single  RndMeth=Simplest
  Data Type Conversion4 : DataTypeConversion  OutDataTypeStr=single  RndMeth=Simplest
  Delay1 : Delay  DelayLength=PI_params.delay_Currents
  Delay2 : Delay  DelayLength=PI_params.delay_Position
  "Get_PU " : Subsystem
  Get_QEP_Counts : Gain  Gain=pmsm.QEPSlits  OutDataTypeStr=uint16  RndMeth=Simplest
  Inverting OpAmp : Gain  Gain=1/PU_System.I_base  OutDataTypeStr=dataType  RndMeth=Simplest
  Selector : Selector  InputPortWidth=3  IndexOptions=Index vector (dialog)  Indices=[1 2]  OutputSizes=1
  Iab_fb : Outport  VectorParamsAs1DForOutWhenUnconnected=off
  Pos_fb : Outport  Port=2  VectorParamsAs1DForOutWhenUnconnected=off
  wires:
  Selector/1 -> Inverting OpAmp/1
  Delay2/1 -> "Get_PU "/1(rad)  "Theta_m"
  Data Type Conversion2/1 -> Delay2/1  "Theta_m"
  Bus Selector/1 -> Data Type Conversion2/1  "<MtrPos>"
  Info/1 -> Bus Selector/1
  PhaseCurr/1 -> Data Type Conversion4/1
  Data Type Conversion4/1 -> Delay1/1
  Delay1/1 -> Selector/1  "Iab_fb"
  "Get_PU "/1(PU) -> Get_QEP_Counts/1
  Inverting OpAmp/1 -> Iab_fb/1
  Get_QEP_Counts/1 -> Pos_fb/1

== system dsPIC33CK256MP508_MCLV2_SMO/Speed Control/Enable Switch/Codegen ==
  note: Toggle between enable and disable on press on Button S2
  Button S2 : MCHP_Blockset/Digital IO/Digital Input  PORT=Dynamic Options  PORT_TXT="D   [ 0 : 15 ]"  PIN=5  PACK=off  SIMULTANEOUS=off  ORDERING=None  SampleTime=-1  MCHP_PORT={Digital In}{DIN}2:0:D5;  MCHP_MASTERLINK=dsPIC33CK256MP508_MCLV2_SMO1/Hardware Init/Microchip Master
      settings: SourceProductName=MPLAB Device Blocks for Simulink
  Triggered Subsystem : Subsystem  TreatAsAtomicUnit=on
  wires:
  Button S2/1 -> Triggered Subsystem/Trigger

== system dsPIC33CK256MP508_MCLV2_SMO/Speed Control/Enable Switch/Sim ==
  Constant : Constant  OutDataTypeStr=Inherit: Inherit via back propagation
  Data Store Write : DataStoreWrite  DataStoreName=Enable  IndexOptions=Index vector (dialog)  Indices=1  OutputSizes=1
  wires:
  Constant/1 -> Data Store Write/1

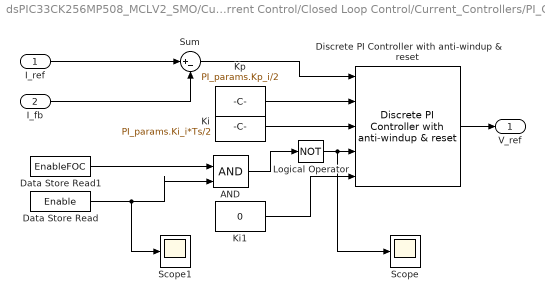
== system dsPIC33CK256MP508_MCLV2_SMO/Current Control/Closed Loop Control/Current_Controllers/PI_Controller_Id ==
  I_ref : Inport
  I_fb : Inport  Port=2
  AND : Logic  IconShape=distinctive  AllPortsSameDT=off  OutDataTypeStr=boolean
  Data Store Read : DataStoreRead  DataStoreName=Enable  IndexOptions=Index vector (dialog)  Indices=1  OutputSizes=1
  Data Store Read1 : DataStoreRead  DataStoreName=EnableFOC  IndexOptions=Index vector (dialog)  Indices=1  OutputSizes=1
  Discrete PI Controller with anti-windup & reset : mcbcontrolslib/Discrete PI Controller  with anti-windup & reset  UpperSaturationLimit=1  LowerSaturationLimit=-1
      settings: SourceProductBaseCode=MT
  Ki : Constant  Value=PI_params.Ki_i*Ts/2  OutDataTypeStr=dataType  SampleTime=-1
  Ki1 : Constant  Value=0  OutDataTypeStr=dataType  SampleTime=-1
  Kp : Constant  Value=PI_params.Kp_i/2  OutDataTypeStr=dataType2  SampleTime=-1
  Logical Operator : Logic  Operator=NOT  IconShape=distinctive  AllPortsSameDT=off  OutDataTypeStr=boolean
  Scope : Scope
  Scope1 : Scope
  Sum : Sum  Inputs=|+-  OutDataTypeStr=Inherit: Same as first input
  V_ref : Outport  VectorParamsAs1DForOutWhenUnconnected=off
  wires:
  I_ref/1 -> Sum/1
  I_fb/1 -> Sum/2
  Data Store Read1/1 -> AND/1
  Discrete PI Controller with anti-windup & reset/1 -> V_ref/1
  Sum/1 -> Discrete PI Controller with anti-windup & reset/1
  Kp/1 -> Discrete PI Controller with anti-windup & reset/2
  Ki/1 -> Discrete PI Controller with anti-windup & reset/3
  Logical Operator/1 -> Scope/1, Discrete PI Controller with anti-windup & reset/4
  Ki1/1 -> Discrete PI Controller with anti-windup & reset/5
  Data Store Read/1 -> Scope1/1, AND/2
  AND/1 -> Logical Operator/1

== system dsPIC33CK256MP508_MCLV2_SMO/Current Control/Closed Loop Control/Current_Controllers/PI_Controller_Iq ==
  I_ref : Inport
  I_fb : Inport  Port=2
  AND : Logic  IconShape=distinctive  AllPortsSameDT=off  OutDataTypeStr=boolean
  Data Store Read : DataStoreRead  DataStoreName=Enable  IndexOptions=Index vector (dialog)  Indices=1  OutputSizes=1
  Data Store Read1 : DataStoreRead  DataStoreName=EnableFOC  IndexOptions=Index vector (dialog)  Indices=1  OutputSizes=1
  Discrete PI Controller with anti-windup & reset : mcbcontrolslib/Discrete PI Controller  with anti-windup & reset  UpperSaturationLimit=1  LowerSaturationLimit=-1
      settings: SourceProductBaseCode=MT
  Ki : Constant  Value=PI_params.Ki_i*Ts/2  OutDataTypeStr=dataType  SampleTime=-1
  Kp : Constant  Value=PI_params.Kp_i/2  OutDataTypeStr=dataType2  SampleTime=-1
  Kp1 : Constant  Value=0  OutDataTypeStr=dataType  SampleTime=-1
  Logical Operator : Logic  Operator=NOT  IconShape=distinctive  AllPortsSameDT=off  OutDataTypeStr=boolean
  Sum : Sum  Inputs=|+-  OutDataTypeStr=Inherit: Same as first input
  V_ref : Outport  VectorParamsAs1DForOutWhenUnconnected=off
  wires:
  Discrete PI Controller with anti-windup & reset/1 -> V_ref/1
  Data Store Read1/1 -> AND/1
  I_fb/1 -> Sum/2
  I_ref/1 -> Sum/1
  Kp/1 -> Discrete PI Controller with anti-windup & reset/2
  Sum/1 -> Discrete PI Controller with anti-windup & reset/1
  Ki/1 -> Discrete PI Controller with anti-windup & reset/3
  Logical Operator/1 -> Discrete PI Controller with anti-windup & reset/4
  Kp1/1 -> Discrete PI Controller with anti-windup & reset/5
  Data Store Read/1 -> AND/2
  AND/1 -> Logical Operator/1

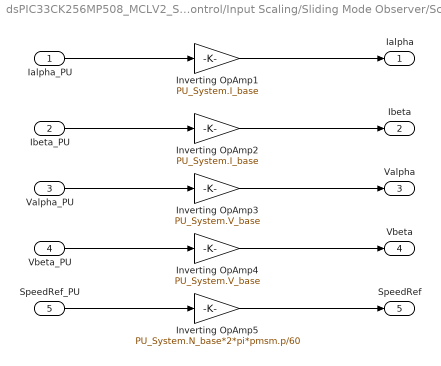
== system dsPIC33CK256MP508_MCLV2_SMO/Current Control/Input Scaling/Sliding Mode Observer/Scaling ==
  Ialpha_PU : Inport
  Ibeta_PU : Inport  Port=2
  Valpha_PU : Inport  Port=3
  Vbeta_PU : Inport  Port=4
  SpeedRef_PU : Inport  Port=5
  Inverting OpAmp1 : Gain  Gain=PU_System.I_base  OutDataTypeStr=fixdt(1,16,12)  RndMeth=Simplest
  Inverting OpAmp2 : Gain  Gain=PU_System.I_base  OutDataTypeStr=fixdt(1,16,12)  RndMeth=Simplest
  Inverting OpAmp3 : Gain  Gain=PU_System.V_base  OutDataTypeStr=fixdt(1,16,11)  RndMeth=Simplest
  Inverting OpAmp4 : Gain  Gain=PU_System.V_base  OutDataTypeStr=fixdt(1,16,11)  RndMeth=Simplest
  Inverting OpAmp5 : Gain  Gain=PU_System.N_base*2*pi*pmsm.p/60  OutDataTypeStr=fixdt(1,16,3)  RndMeth=Simplest
  Ialpha : Outport
  Ibeta : Outport  Port=2
  Valpha : Outport  Port=3
  Vbeta : Outport  Port=4
  SpeedRef : Outport  Port=5
  wires:
  Vbeta_PU/1 -> Inverting OpAmp4/1
  SpeedRef_PU/1 -> Inverting OpAmp5/1
  Inverting OpAmp2/1 -> Ibeta/1
  Inverting OpAmp3/1 -> Valpha/1
  Ibeta_PU/1 -> Inverting OpAmp2/1
  Inverting OpAmp4/1 -> Vbeta/1
  Ialpha_PU/1 -> Inverting OpAmp1/1
  Inverting OpAmp1/1 -> Ialpha/1
  Valpha_PU/1 -> Inverting OpAmp3/1
  Inverting OpAmp5/1 -> SpeedRef/1

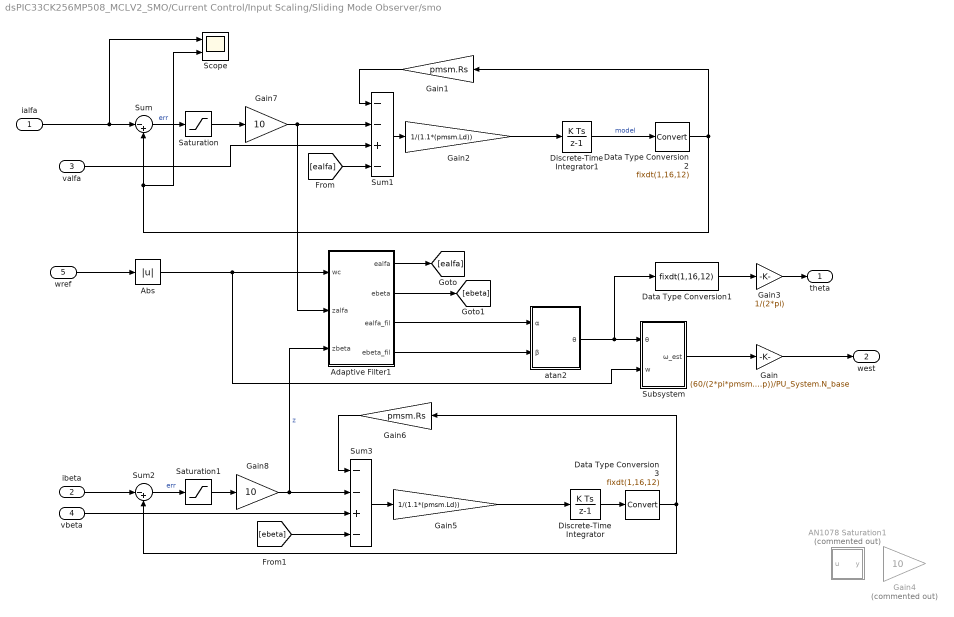
== system dsPIC33CK256MP508_MCLV2_SMO/Current Control/Input Scaling/Sliding Mode Observer/smo ==
  ialfa : Inport
  ibeta : Inport  Port=2
  valfa : Inport  Port=3
  vbeta : Inport  Port=4
  wref : Inport  Port=5
  AN1078 Saturation1 : MATLAB Function  Commented=on  TreatAsAtomicUnit=on
  Abs : Abs
  Adaptive Filter1 : Subsystem
  Data Type Conversion1 : DataTypeConversion  OutDataTypeStr=fixdt(1,16,12)
  Data Type Conversion2 : DataTypeConversion  OutDataTypeStr=fixdt(1,16,12)
  Data Type Conversion3 : DataTypeConversion  OutDataTypeStr=fixdt(1,16,12)
  Discrete-Time Integrator : DiscreteIntegrator  SampleTime=-1  OutDataTypeStr=fixdt(1,32,17)  ICPrevOutput=DiscIntNeverNeededParam  ICPrevScaledInput=DiscIntNeverNeededParam
  Discrete-Time Integrator1 : DiscreteIntegrator  SampleTime=-1  OutDataTypeStr=fixdt(1,32,17)  ICPrevOutput=DiscIntNeverNeededParam  ICPrevScaledInput=DiscIntNeverNeededParam
  Gain : Gain  Gain=(60/(2*pi*pmsm.p))/PU_System.N_base  OutDataTypeStr=dataType
  Gain1 : Gain  Gain=pmsm.Rs  OutDataTypeStr=fixdt(1,16,12)
  Gain2 : Gain  Gain=1/(1.1*(pmsm.Ld))  OutDataTypeStr=fixdt(1,32,14)
  Gain3 : Gain  Gain=1/(2*pi)  OutDataTypeStr=dataType
  Gain4 : Gain  Commented=on  Gain=10
  Gain5 : Gain  Gain=1/(1.1*(pmsm.Ld))  OutDataTypeStr=fixdt(1,32,14)
  Gain6 : Gain  Gain=pmsm.Rs  OutDataTypeStr=fixdt(1,16,12)
  Gain7 : Gain  Gain=10  OutDataTypeStr=fixdt(1,16,8)
  Gain8 : Gain  Gain=10  OutDataTypeStr=fixdt(1,16,8)
  Saturation : Saturate
  Saturation1 : Saturate
  Scope : Scope  NumInputPorts=2
  Subsystem : Subsystem
  Sum : Sum  Inputs=|-+
  Sum1 : Sum  Inputs=--+-  AccumDataTypeStr=fixdt(1,32,17)
  Sum2 : Sum  Inputs=|-+
  Sum3 : Sum  Inputs=--+-
  atan2 : Subsystem
  theta : Outport  VectorParamsAs1DForOutWhenUnconnected=off
  west : Outport  Port=2  VectorParamsAs1DForOutWhenUnconnected=off
  wires:
  atan2/1(θ) -> Data Type Conversion1/1, Subsystem/1(θ)
  Discrete-Time Integrator1/1 -> Data Type Conversion2/1  "model"
  ialfa/1 -> Scope/1, Sum/1
  Sum/1 -> Saturation/1  "err"
  Sum1/1 -> Gain2/1
  Gain2/1 -> Discrete-Time Integrator1/1
  Gain7/1 -> Sum1/2, Adaptive Filter1/2(zalfa)
  Subsystem/1(ω_est) -> Gain/1
  Sum2/1 -> Saturation1/1  "err"
  ibeta/1 -> Sum2/1
  Sum3/1 -> Gain5/1
  Gain5/1 -> Discrete-Time Integrator/1
  Gain8/1 -> Adaptive Filter1/3(zbeta), Sum3/2  "z"
  Discrete-Time Integrator/1 -> Data Type Conversion3/1
  vbeta/1 -> Sum3/3
  Gain6/1 -> Sum3/1
  Gain1/1 -> Sum1/1
  valfa/1 -> Sum1/3
  wref/1 -> Abs/1
  Adaptive Filter1/1(ealfa) -> [ealfa]
  Saturation/1 -> Gain7/1
  Saturation1/1 -> Gain8/1
  Adaptive Filter1/2(ebeta) -> [ebeta]
  [ealfa] -> Sum1/4
  [ebeta] -> Sum3/4
  Adaptive Filter1/3(ealfa_fil) -> atan2/1(α)
  Adaptive Filter1/4(ebeta_fil) -> atan2/2(β)
  Data Type Conversion1/1 -> Gain3/1
  Data Type Conversion2/1 -> Gain1/1, Scope/2, Sum/2
  Data Type Conversion3/1 -> Gain6/1, Sum2/2
  Gain/1 -> west/1
  Abs/1 -> Subsystem/2(w), Adaptive Filter1/1(wc)
  Gain3/1 -> theta/1

== system dsPIC33CK256MP508_MCLV2_SMO/Current Control/Output Scaling/Mode Selector/Subsystem1 ==
  Count : Inport
  AND : Logic  IconShape=distinctive  AllPortsSameDT=off  OutDataTypeStr=boolean
  Compare To Constant : simulink/Logic and Bit Operations/Compare To Constant  relop=>=  const=2  OutDataTypeStr=boolean
  Compare To Constant1 : simulink/Logic and Bit Operations/Compare To Constant  relop=<  const=1  OutDataTypeStr=boolean
  Compare To Constant2 : simulink/Logic and Bit Operations/Compare To Constant  relop=<  const=2  OutDataTypeStr=boolean
  Compare To Constant3 : simulink/Logic and Bit Operations/Compare To Constant  relop=>  const=1  OutDataTypeStr=boolean
  Data Store Write : DataStoreWrite  DataStoreName=EnCurOffset  IndexOptions=Index vector (dialog)  Indices=1  OutputSizes=1
  Data Store Write1 : DataStoreWrite  DataStoreName=EnableFOC  IndexOptions=Index vector (dialog)  Indices=1  OutputSizes=1
  Data Store Write2 : DataStoreWrite  DataStoreName=EnPosOffset  IndexOptions=Index vector (dialog)  Indices=1  OutputSizes=1
  Gain : Gain  Gain=1/PWM_frequency  OutDataTypeStr=dataType2  RndMeth=Simplest
  Current Offset : Outport
  PositionOffset : Outport  Port=2
  EnableFOC : Outport  Port=3
  wires:
  Count/1 -> Gain/1
  Gain/1 -> Compare To Constant1/1, Compare To Constant3/1, Compare To Constant2/1, Compare To Constant/1
  Compare To Constant/1 -> Data Store Write1/1, EnableFOC/1
  Compare To Constant1/1 -> Data Store Write/1, Current Offset/1
  Compare To Constant2/1 -> AND/2
  Compare To Constant3/1 -> AND/1
  AND/1 -> Data Store Write2/1, PositionOffset/1

== system dsPIC33CK256MP508_MCLV2_SMO/Current Control/Output Scaling/Mode Selector/Up Counter ==
  Enable : EnablePort  StatesWhenEnabling=reset
  Add1 : Sum  SaturateOnIntegerOverflow=on
  Constant : Constant  OutDataTypeStr=uint32
  Delay : Delay  DelayLength=1
  Count : Outport  InitialOutput=0
  wires:
  Delay/1 -> Add1/2
  Add1/1 -> Count/1, Delay/1
  Constant/1 -> Add1/1

== system dsPIC33CK256MP508_MCLV2_SMO/Current Control/Serial Tx/UART_TX/Debug_Data ==
  Count : Inport
  Data : Inport  Port=2
  Bitwise Operator2 : simulink/Logic and Bit Operations/Bitwise Operator  logicop=AND  UseBitMask=on  BitMask=bin2dec('0000000011111111')  BitMaskRealWorld=Stored Integer
  Bitwise Operator3 : simulink/Logic and Bit Operations/Bitwise Operator  logicop=AND  UseBitMask=on  BitMask=bin2dec('0000000011111111')  BitMaskRealWorld=Stored Integer
  Data Type Conversion1 : DataTypeConversion  OutDataTypeStr=uint8  RndMeth=Simplest
  Data Type Conversion2 : DataTypeConversion  OutDataTypeStr=uint8  RndMeth=Simplest
  Data Type Conversion3 : DataTypeConversion  OutDataTypeStr=uint16  ConvertRealWorld=Stored Integer (SI)  RndMeth=Simplest
  Mux : Mux  Inputs=3
  Shift Arithmetic2 : ArithShift  BitShiftNumber=8  BitShiftDirection=Right
  Data_log : Outport
  wires:
  Mux/1 -> Data_log/1
  Data/1 -> Data Type Conversion3/1
  Count/1 -> Mux/1
  Bitwise Operator2/1 -> Data Type Conversion1/1
  Shift Arithmetic2/1 -> Bitwise Operator3/1
  Bitwise Operator3/1 -> Data Type Conversion2/1
  Data Type Conversion3/1 -> Bitwise Operator2/1, Shift Arithmetic2/1
  Data Type Conversion1/1 -> Mux/2
  Data Type Conversion2/1 -> Mux/3

== system dsPIC33CK256MP508_MCLV2_SMO/Current Control/Serial Tx/UART_TX/SCI_Tx ==
  Data_Log : Inport
  End : Constant  Value=hex2dec('45')  OutDataTypeStr=uint8
  Mux : Mux  Inputs=3
  Start : Constant  Value=hex2dec('53')  OutDataTypeStr=uint8
  UART Tx : MCHP_Blockset/BUS UART/UART Tx  UART_REF=2  ORDERING=None  AllOrNothing=off  SampleTime=-1  MCHP_MASTERLINK=dsPIC33CK256MP508_MCLV2_SMO1/Hardware Init/Microchip Master  NSend_Input=off  UART_String=off  NSend_Output=off
      settings: SourceProductName=MPLAB Device Blocks for Simulink
  wires:
  Mux/1 -> UART Tx/1
  Data_Log/1 -> Mux/2
  Start/1 -> Mux/1
  End/1 -> Mux/3

== system dsPIC33CK256MP508_MCLV2_SMO/Inverter and Motor/Simulation/Sensor_Measurements/Get_PU  ==
  rad : Inport
  Constant2 : Constant  Value=2*pi  OutDataTypeStr=single  SampleTime=-1
  Get_PU : Gain  Gain=1/(2*pi)  OutDataTypeStr=dataType  RndMeth=Simplest
  Mod : Math  Operator=mod  SaturateOnIntegerOverflow=on
  PU : Outport  VectorParamsAs1DForOutWhenUnconnected=off
  wires:
  Mod/1 -> Get_PU/1
  Constant2/1 -> Mod/2
  rad/1 -> Mod/1
  Get_PU/1 -> PU/1

== system dsPIC33CK256MP508_MCLV2_SMO/Speed Control/Enable Switch/Codegen/Triggered Subsystem ==
  Trigger : TriggerPort  TriggerType=falling  VariantControl=Variant
  Data Store Write : DataStoreWrite  DataStoreName=Enable  IndexOptions=Index vector (dialog)  Indices=1  OutputSizes=1
  Delay : Delay  DelayLength=1  InitialCondition=0
  NOT : Logic  Operator=NOT  IconShape=distinctive  AllPortsSameDT=off  OutDataTypeStr=boolean
  wires:
  NOT/1 -> Data Store Write/1, Delay/1
  Delay/1 -> NOT/1

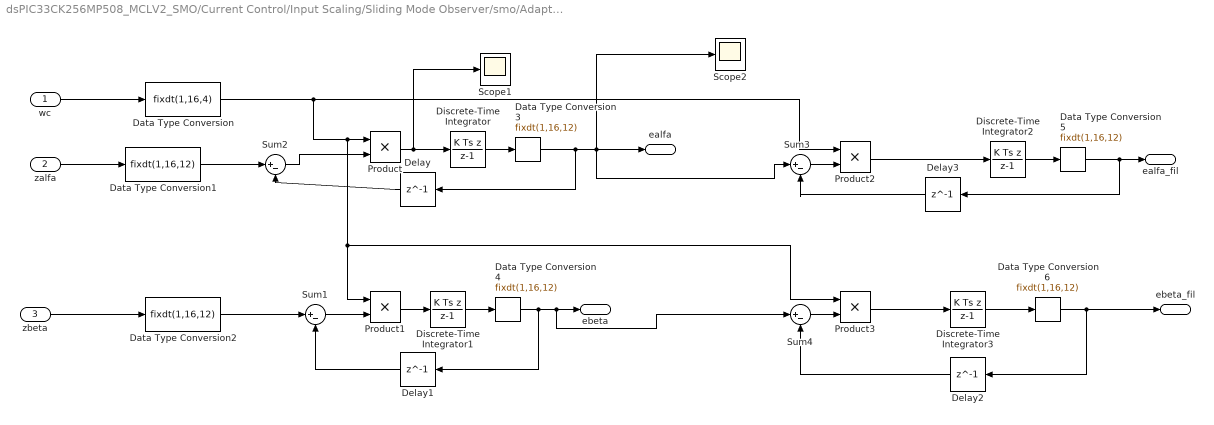
== system dsPIC33CK256MP508_MCLV2_SMO/Current Control/Input Scaling/Sliding Mode Observer/smo/Adaptive Filter1 ==
  wc : Inport
  zalfa : Inport  Port=2
  zbeta : Inport  Port=3
  Data Type Conversion : DataTypeConversion  OutDataTypeStr=fixdt(1,16,4)
  Data Type Conversion{1..6} (6 alike) : DataTypeConversion  OutDataTypeStr=fixdt(1,16,12)
  Delay{,1..3} (4 alike) : Delay  DelayLength=1
  Discrete-Time Integrator{,1..3} (4 alike) : DiscreteIntegrator  IntegratorMethod=Integration: Backward Euler  SampleTime=-1  OutDataTypeStr=fixdt(1,32,17)  ICPrevOutput=DiscIntNeverNeededParam  ICPrevScaledInput=DiscIntNeverNeededParam
  Product : Product  OutDataTypeStr=fixdt(1,32,17)
  Product1 : Product  OutDataTypeStr=fixdt(1,32,17)
  Product2 : Product
  Product3 : Product
  Scope1 : Scope
  Scope2 : Scope
  Sum{1..4} (4 alike) : Sum  Inputs=|+-
  ealfa : Outport  VectorParamsAs1DForOutWhenUnconnected=off
  ebeta : Outport  Port=2  VectorParamsAs1DForOutWhenUnconnected=off
  ealfa_fil : Outport  Port=3  VectorParamsAs1DForOutWhenUnconnected=off
  ebeta_fil : Outport  Port=4  VectorParamsAs1DForOutWhenUnconnected=off
  wires:
  Sum2/1 -> Product/2
  Product/1 -> Discrete-Time Integrator/1, Scope1/1
  zalfa/1 -> Data Type Conversion1/1
  wc/1 -> Data Type Conversion/1
  Product1/1 -> Discrete-Time Integrator1/1
  Sum1/1 -> Product1/2
  zbeta/1 -> Data Type Conversion2/1
  Discrete-Time Integrator1/1 -> Data Type Conversion4/1
  Product2/1 -> Discrete-Time Integrator2/1
  Sum3/1 -> Product2/2
  Discrete-Time Integrator2/1 -> Data Type Conversion5/1
  Discrete-Time Integrator3/1 -> Data Type Conversion6/1
  Sum4/1 -> Product3/2
  Product3/1 -> Discrete-Time Integrator3/1
  Data Type Conversion/1 -> Product3/1, Product1/1, Product/1, Product2/1
  Data Type Conversion1/1 -> Sum2/1
  Data Type Conversion2/1 -> Sum1/1
  Discrete-Time Integrator/1 -> Data Type Conversion3/1
  Data Type Conversion3/1 -> Delay/1, Scope2/1, Sum3/1, ealfa/1
  Data Type Conversion4/1 -> Delay1/1, Sum4/1, ebeta/1
  Delay/1 -> Sum2/2
  Delay1/1 -> Sum1/2
  Delay2/1 -> Sum4/2
  Delay3/1 -> Sum3/2
  Data Type Conversion5/1 -> ealfa_fil/1, Delay3/1
  Data Type Conversion6/1 -> ebeta_fil/1, Delay2/1

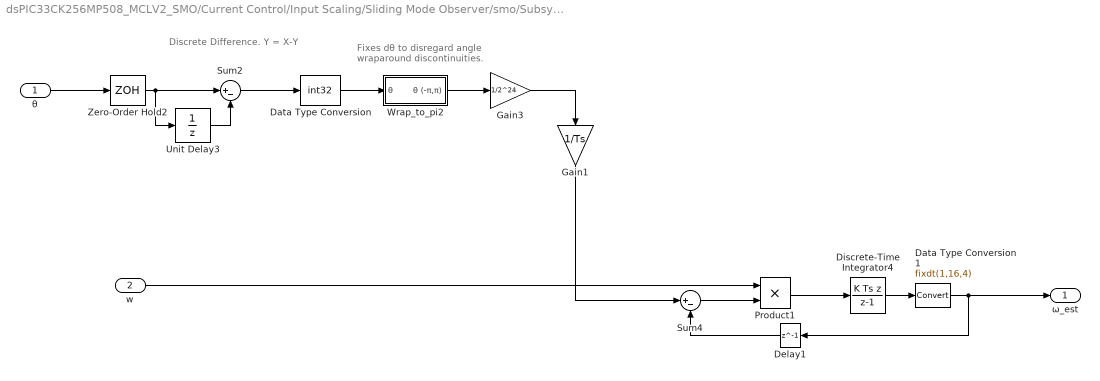
== system dsPIC33CK256MP508_MCLV2_SMO/Current Control/Input Scaling/Sliding Mode Observer/smo/Subsystem ==
  note: Discrete
      | Difference.
      | Y = X-Y
  note: Fixes dθ to disregard angle
      | wraparound discontinuities.
  θ : Inport
  w : Inport  Port=2
  Data Type Conversion : DataTypeConversion  OutDataTypeStr=int32  ConvertRealWorld=Stored Integer (SI)
  Data Type Conversion1 : DataTypeConversion  OutDataTypeStr=fixdt(1,16,4)
  Delay1 : Delay  DelayLength=1
  Discrete-Time Integrator4 : DiscreteIntegrator  IntegratorMethod=Integration: Backward Euler  SampleTime=-1  OutDataTypeStr=fixdt(1,32,8)  ICPrevOutput=DiscIntNeverNeededParam  ICPrevScaledInput=DiscIntNeverNeededParam
  Gain1 : Gain  Gain=1/Ts  OutDataTypeStr=fixdt(1,16,3)
  Gain3 : Gain  Gain=1/2^24  OutDataTypeStr=fixdt(1,16,12)
  Product1 : Product  OutDataTypeStr=fixdt(1,32,8)
  Sum2 : Sum  Inputs=|+-  AccumDataTypeStr=fixdt(1,16,12)  OutDataTypeStr=fixdt(1,32,24)
  Sum4 : Sum  Inputs=|+-
  Unit Delay3 : UnitDelay  SampleTime=Ts  HasFrameUpgradeWarning=on
  Wrap_to_pi2 : Subsystem  VariantControl=VSS_STD
  Zero-Order Hold2 : ZeroOrderHold  SampleTime=Ts
  ω_est : Outport  VectorParamsAs1DForOutWhenUnconnected=off
  wires:
  Unit Delay3/1 -> Sum2/2
  Zero-Order Hold2/1 -> Sum2/1, Unit Delay3/1
  Wrap_to_pi2/1(θ (-π,π)) -> Gain3/1
  Sum4/1 -> Product1/2
  Discrete-Time Integrator4/1 -> Data Type Conversion1/1
  Product1/1 -> Discrete-Time Integrator4/1
  θ/1 -> Zero-Order Hold2/1
  Gain1/1 -> Sum4/1
  Delay1/1 -> Sum4/2
  Sum2/1 -> Data Type Conversion/1
  Data Type Conversion/1 -> Wrap_to_pi2/1(θ)
  Gain3/1 -> Gain1/1
  Data Type Conversion1/1 -> Delay1/1, ω_est/1
  w/1 -> Product1/1

== system dsPIC33CK256MP508_MCLV2_SMO/Current Control/Input Scaling/Sliding Mode Observer/smo/atan2 ==
  note: Consistent with Microchip notation:
      |
      | x_α = cos(θ) * x_d - sin(θ) * x_q
      | x_β = sin(θ) * x_d + cos(θ) * x_q
      |
      | θ = atan2(sin(θ)/cos(θ)) = atan2(-x_α/x_β)
      |
      | provided x_d = 0, which is true in case of E_d
  α : Inport
  β : Inport  Port=2
  Bias2 : Bias  Bias=(pi/4)-(pi/25)
  Data Type Conversion3 : DataTypeConversion  OutDataTypeStr=fixdt(1,16,12)
  Data Type Conversion4 : DataTypeConversion  OutDataTypeStr=uint16  ConvertRealWorld=Stored Integer (SI)
  Gain2 : Gain  Gain=1/2^12  OutDataTypeStr=fixdt(1,16,12)
  Gain3 : Gain  Gain=-1  OutDataTypeStr=Inherit: Same as input
  Subsystem1 : Subsystem
  Trigonometric Function : Trigonometry  Operator=atan2  ApproximationMethod=CORDIC
  Wrap_to_pi1 : Subsystem  VariantControl=VSS_STD
  θ : Outport  VectorParamsAs1DForOutWhenUnconnected=off
  wires:
  Trigonometric Function/1 -> Data Type Conversion3/1
  Gain3/1 -> Trigonometric Function/1
  α/1 -> Gain3/1
  β/1 -> Trigonometric Function/2
  Data Type Conversion3/1 -> Subsystem1/1(theta(-pi,pi))
  Subsystem1/1(theta(0,2pi)) -> Bias2/1
  Bias2/1 -> Data Type Conversion4/1
  Data Type Conversion4/1 -> Wrap_to_pi1/1(θ)
  Wrap_to_pi1/1(θ (0,2π)) -> Gain2/1  "z"
  Gain2/1 -> θ/1

== system dsPIC33CK256MP508_MCLV2_SMO/Current Control/Input Scaling/Sliding Mode Observer/smo/Subsystem/Wrap_to_pi2 ==
  note: What's left after
      | division by 2pi
  note: This block limits the output angle between +/- π.
  note: Add pi
  note: What's left after
      | division by 2pi
      | again
  note: Subtract pi
  θ : Inport
  Bias : Bias  Bias=pi*16777216
  Bias1 : Bias  Bias=-pi*16777216
  Math Function : Math  Operator=mod  SignedPower=on  SaturateOnIntegerOverflow=on
  Math Function1 : Math  Operator=mod  SignedPower=on  SaturateOnIntegerOverflow=on
  load torque1 : Constant  Value=2*pi*16777216  OutDataTypeStr=int32  SampleTime=Ts
  θ (-π,π) : Outport  VectorParamsAs1DForOutWhenUnconnected=off
  wires:
  Math Function1/1 -> Bias/1
  θ/1 -> Math Function1/1
  Math Function/1 -> Bias1/1
  load torque1/1 -> Math Function1/2, Math Function/2
  Bias/1 -> Math Function/1
  Bias1/1 -> θ (-π,π)/1

== system dsPIC33CK256MP508_MCLV2_SMO/Current Control/Input Scaling/Sliding Mode Observer/smo/atan2/Subsystem1 ==
  theta(-pi,pi) : Inport
  2pi : Constant  Value=2*pi  OutDataTypeStr=fixdt(1,16,12)  SampleTime=Ts  mask(TL_Constant){data={'date',734873.5078369329}}
      settings: CopyFcn=if exist('tl_reset_reviewflag','file')==2,tl_reset_reviewflag(gcbh);end  DeleteFcn=if exist('delete_tlblock','file')==2,delete_tlblock(gcbh);end  NameChangeFcn=if exist('rename_tlblock','file')==2,rename_tlblock(gcbh);end  OpenFcn=if exist('tl_open_blockdlg','file')==2,tl_open_blockdlg(gcbh);else,open_system(gcbh,'parameter');end
      mask Help: eval(['if exist(''tl_online_help'',''file'') == 2, tl_online_help(''Topic'',''TL_Constant''),else, web([''jar:file:///'',matlabroot,''/help/toolbox/simulink/help.jar!/slref/' lower(get_param(gcbh,'Blocktype')) '.html''], ''-helpbrowser''),end'])
      mask Display: plot([-0.05, 1.05, NaN, -0.05, 1.05],[.01, .01, NaN, .99, .99])
  Sum : Sum
  Switch2 : Switch  Criteria=u2 > Threshold
  theta(0,2pi) : Outport  VectorParamsAs1DForOutWhenUnconnected=off
  wires:
  2pi/1 -> Sum/2
  theta(-pi,pi)/1 -> Sum/1, Switch2/2, Switch2/1
  Sum/1 -> Switch2/3  "err"
  Switch2/1 -> theta(0,2pi)/1

== system dsPIC33CK256MP508_MCLV2_SMO/Current Control/Input Scaling/Sliding Mode Observer/smo/atan2/Wrap_to_pi1 ==
  note: This block limits the output angle between 0 to 2π.
  θ : Inport
  Math Function : Math  Operator=rem  SignedPower=on  SaturateOnIntegerOverflow=on
  load torque2 : Constant  Value=2*pi*2^12  OutDataTypeStr=uint16  SampleTime=Ts
  θ (0,2π) : Outport  VectorParamsAs1DForOutWhenUnconnected=off
  wires:
  Math Function/1 -> θ (0,2π)/1
  θ/1 -> Math Function/1
  load torque2/1 -> Math Function/2

== stateflow chart dsPIC33CK256MP508_MCLV2_SMO/Current Control/Input Scaling/OpentoClosed/Chart ==
  state Init
    during: Mode = 0;
    SpeedCtrl = 0;
  state Align
    during: Mode = 0;
    SpeedCtrl = 0;
  state ClosedLoopFilter
    during: Mode = 2;
    SpeedCtrl = 1;
  state ClosedLoop
    during: Mode = 2;
    SpeedCtrl = 0;
  state OpenLoop
    during: Mode = 1;
    SpeedCtrl = 0;
  (default) -> Init
  ClosedLoopFilter -> Init : [En == 0]
  ClosedLoop -> Init [order 1] : [En == 0]
  Init -> Align : [En == 1]
  Align -> Init [order 1] : [En == 0]
  OpenLoop -> Init [order 2] : [En == 0]
  Align -> OpenLoop [order 2] : after(0.5,sec)
  ClosedLoop -> ClosedLoopFilter [order 2] : after(0.1,sec)
  OpenLoop -> ClosedLoop [order 1] : after(2,sec)[SpeedFb > Limit]
  data: Limit input fixdt(1,16,14); SpeedFb input fixdt(1,16,14); Mode output uint16; En input boolean; SpeedCtrl output uint16
